simulink subsystem "SCIOutAbstractionMotorSwap"  (R2024b)
settings: Solver=VariableStepAuto  StartTime=0.0  StopTime=10.0  RelTol=1e-3
libraries: svdutilitieslib x1, simulink x1
settings Model: Creator=The MathWorks, Inc.  LastModifiedBy=snarayan
settings RTWCC: GPUComputeCapability=3.5

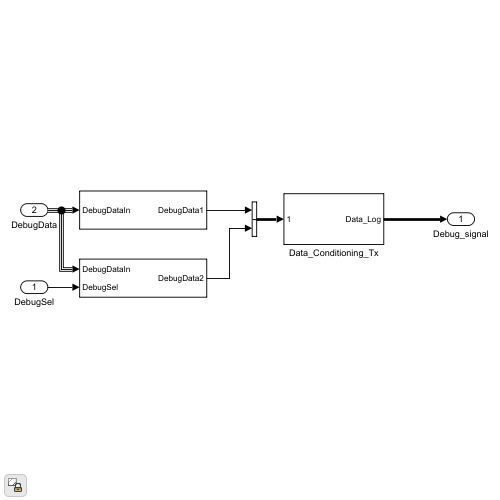
[thumbnail: Simulink's stored preview of the top-level diagram]
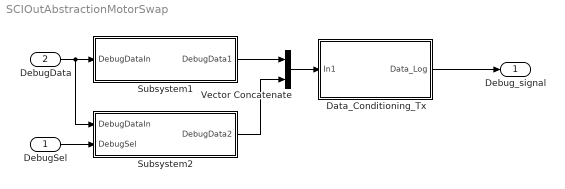
== system SCIOutAbstractionMotorSwap ==
  DebugSel : Inport
  DebugData : Inport  Port=2
  Data_Conditioning_Tx : Subsystem  VariantControl=~isequal(dataType,'single')
  Subsystem1 : Subsystem
  Subsystem2 : Subsystem
  Vector Concatenate : Concatenate
  Debug_signal : Outport
  wires:
  Data_Conditioning_Tx/1(Data_Log) -> Debug_signal/1
  Vector Concatenate/1 -> Data_Conditioning_Tx/1(In1)
  Subsystem1/1(DebugData1) -> Vector Concatenate/1
  DebugData/1 -> Subsystem1/1(DebugDataIn), Subsystem2/1(DebugDataIn)
  DebugSel/1 -> Subsystem2/2(DebugSel)
  Subsystem2/1(DebugData2) -> Vector Concatenate/2

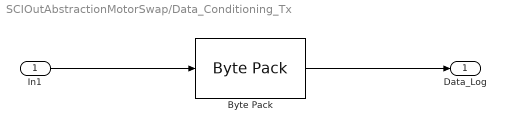
== system SCIOutAbstractionMotorSwap/Data_Conditioning_Tx ==
  In1 : Inport
  Byte Pack : svdutilitieslib/Byte Pack  maskPackedDataType=uint32  datatypes={'single'}  byteAlign=4  blockPlatform=tic2000
  Data_Log : Outport
  wires:
  In1/1 -> Byte Pack/1
  Byte Pack/1 -> Data_Log/1

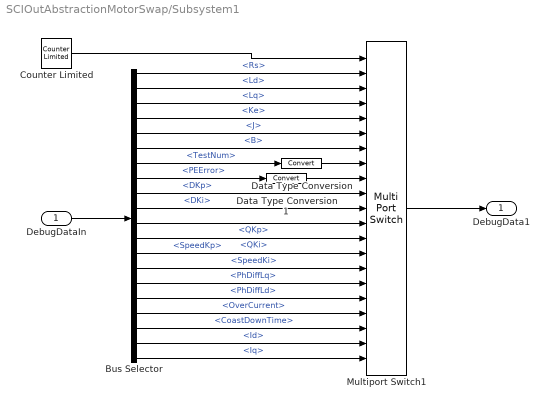
== system SCIOutAbstractionMotorSwap/Subsystem1 ==
  DebugDataIn : Inport
  Bus Selector : BusSelector  OutputSignals=Rs,Ld,Lq,Ke,J,B,TestNum,PEError,DKp,DKi,QKp,QKi,SpeedKp,SpeedKi,PhDiffLq,PhDiffLd,OverCurrent,CoastDownTime,Id,Iq
  Counter Limited : simulink/Sources/Counter Limited  uplimit=19  tsamp=Ts_serialOut
  Data Type Conversion : DataTypeConversion  SaturateOnIntegerOverflow=off  RndMeth=Floor
  Data Type Conversion1 : DataTypeConversion  SaturateOnIntegerOverflow=off  RndMeth=Floor
  Multiport Switch1 : MultiPortSwitch  DataPortOrder=Zero-based contiguous  Inputs=20  DiagnosticForDefault=None  zeroidx=on  SaturateOnIntegerOverflow=off  InputSameDT=off
  DebugData1 : Outport
  wires:
  Bus Selector/10 -> Multiport Switch1/11  "<DKi>"
  Bus Selector/9 -> Multiport Switch1/10  "<DKp>"
  Bus Selector/11 -> Multiport Switch1/12  "<QKp>"
  Bus Selector/12 -> Multiport Switch1/13  "<QKi>"
  Bus Selector/20 -> Multiport Switch1/21  "<Iq>"
  Bus Selector/19 -> Multiport Switch1/20  "<Id>"
  Bus Selector/18 -> Multiport Switch1/19  "<CoastDownTime>"
  Bus Selector/17 -> Multiport Switch1/18  "<OverCurrent>"
  Bus Selector/16 -> Multiport Switch1/17  "<PhDiffLd>"
  Bus Selector/15 -> Multiport Switch1/16  "<PhDiffLq>"
  Bus Selector/14 -> Multiport Switch1/15  "<SpeedKi>"
  Bus Selector/13 -> Multiport Switch1/14  "<SpeedKp>"
  Bus Selector/8 -> Data Type Conversion1/1  "<PEError>"
  Data Type Conversion1/1 -> Multiport Switch1/9
  Bus Selector/7 -> Data Type Conversion/1  "<TestNum>"
  Data Type Conversion/1 -> Multiport Switch1/8
  Bus Selector/3 -> Multiport Switch1/4  "<Lq>"
  Bus Selector/2 -> Multiport Switch1/3  "<Ld>"
  Bus Selector/1 -> Multiport Switch1/2  "<Rs>"
  DebugDataIn/1 -> Bus Selector/1
  Bus Selector/4 -> Multiport Switch1/5  "<Ke>"
  Bus Selector/5 -> Multiport Switch1/6  "<J>"
  Counter Limited/1 -> Multiport Switch1/1
  Multiport Switch1/1 -> DebugData1/1
  Bus Selector/6 -> Multiport Switch1/7  "<B>"

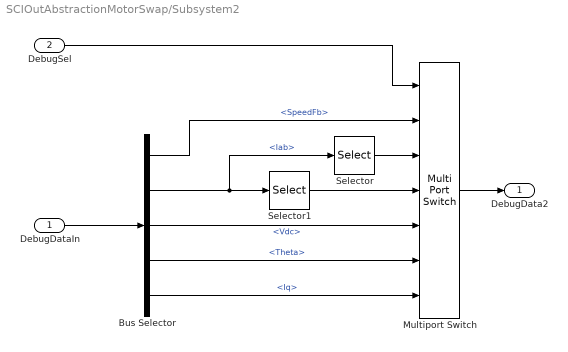
== system SCIOutAbstractionMotorSwap/Subsystem2 ==
  DebugDataIn : Inport
  DebugSel : Inport  Port=2
  Bus Selector : BusSelector  OutputSignals=SpeedFb,Iab,Vdc,Theta,Iq
  Multiport Switch : MultiPortSwitch  Inputs=6  DiagnosticForDefault=None  SaturateOnIntegerOverflow=off  InputSameDT=off
  Selector : Selector  InputPortWidth=3  IndexOptions=Index vector (dialog)  Indices=[1]  OutputSizes=1
  Selector1 : Selector  InputPortWidth=3  IndexOptions=Index vector (dialog)  Indices=[2]  OutputSizes=1
  DebugData2 : Outport
  wires:
  Bus Selector/5 -> Multiport Switch/7  "<Iq>"
  Bus Selector/4 -> Multiport Switch/6  "<Theta>"
  Selector1/1 -> Multiport Switch/4
  Bus Selector/3 -> Multiport Switch/5  "<Vdc>"
  Selector/1 -> Multiport Switch/3
  Bus Selector/2 -> Selector1/1, Selector/1  "<Iab>"
  Bus Selector/1 -> Multiport Switch/2  "<SpeedFb>"
  DebugDataIn/1 -> Bus Selector/1
  Multiport Switch/1 -> DebugData2/1
  DebugSel/1 -> Multiport Switch/1
